simulink model "MSREPrimaryLoop_PlantLevel"  (R2024a)
settings: Solver=VariableStepAuto  StartTime=0.0  StopTime=500000  MaxStep=0.1  RelTol=1e-3
undefined symbols (not defined in the file): a_f, a_g, axialFuelImportance, axialGraphiteImportance, axialPowerFraction, beta, beta_t, bubbleSaturationLevel, bypassRatio, C0, coolantPHXChannelLength, coolantPHXDh, coolantPHXFlowArea, coreCorrectionNominalFlowRate, coreDowncomerArea, coreDowncomerHydraulicDiameter, coreDowncomerLength, coreDowncomerVolume, coreFlowArea, coreFuelVolume, coreInletFlowDistributerArea, coreInletFlowDistributerHydralicDiameter, coreInletFlowDistributerLength, coreInletFlowDistributerVolume, coreLowerPlenumArea, coreLowerPlenumHydraulicDiameter, coreLowerPlenumLength, coreLowerPlenumVolume, coreUpperPlenumArea, coreUpperPlenumLength, coreUpperPlenumVolume, coreVolume, cpGraphite, day, decayScale, decaySSFraction, dissolusionRatio, dMin, dScale, dsmConst, DXeG, externalReactivity, Fiss_factor, fuelChannelHydrualicDiameter, fuelChannelLength, fuelDepositRatio, fuelFraction, fuelGraphiteArea, fuelGraphiteHeatTransferCoefficient, gamma0, gamma1, gamma2, gasExchangeRatio, gasMixingEfficiency, gasPurgeRate, gasStrippingEfficiency, graphiteKDiff, graphiteUnitCellThickness, initialIodineConcentration, InitialXeMolarConcentration ... (+66)
libraries: fl_lib x291, nesl_utility x101, SimscapeFluids_lib x24, simulink x5, slpidlib x1
(part 10 of 13)

== system MSREPrimaryLoop_PlantLevel/Pump MSRE/Pump/PumpIdeal/XenonCalcPump/InterphaseTranfser ==
  note: This local to volume isn't strick. Either add an integral or reduce the length of the node if variation is large.
  CxSalt : Inport
  GasRef : Inport  Port=2
  CxGas : Inport  Port=3
  Constitutive : Subsystem
  MixtureVolume : Gain  Gain=PipeVolume
  Subsystem1 : Subsystem  ReferencedSubsystem=GasToAlpha
  Transfer Term : MATLAB Function  TreatAsAtomicUnit=on
  Ref : PMIOPort  Side=Left
  TranfserRate : Outport
  wires:
  Transfer Term/1(volRate) -> MixtureVolume/1
  MixtureVolume/1 -> TranfserRate/1
  Constitutive/3(k) -> Transfer Term/6(k)
  Constitutive/2(dsm) -> Transfer Term/5(dsm)
  GasRef/1 -> Subsystem1/1
  Subsystem1/1 -> Transfer Term/3(alpha)
  Constitutive/1(K) -> Transfer Term/4(K)
  CxSalt/1 -> Transfer Term/1(CxS)
  CxGas/1 -> Transfer Term/2(CxG)
  connections:
  Constitutive/LConn1 -- Ref/RConn1

== system MSREPrimaryLoop_PlantLevel/Pump MSRE/Pump/PumpIdeal/XenonCalcPump/Salt ==
  XeLIn : Inport  PortDimensions=1
  IodineSNumberDensity : Inport  Port=2  PortDimensions=1
  T_f_ave : Inport  Port=3
  GasRef : Inport  Port=4  PortDimensions=1
  VolumeRate : Inport  Port=5
  Interphase : Inport  Port=6
  Add : Sum  Inputs=+++--  InputSameDT=on
  Decay : Gain  Gain=xeDecayConstant
  InPipeGeneration : Subsystem
      settings: PortSchema="{\"entries\":[{\"content\":{\"sides\":[{\"content\":{\"connectorIds\":[\"In1\"]},\"type\":\"ConnectorPlacement.EquallySpacedRectSide\",\"uuid\":\"cf58f9e2-4051-4ec0-bfd5-a375f3464f67\"},{\"content\":{\"connectorIds\":[\"Out1\"],\"side\":\"RIGHT\"},\"type\":\"ConnectorPlacement.EquallySpacedRectSide\",\"uuid\":\"cf475b22-0422-4ebc-b148-ab559744c6ba\"},{\"content\":{\"connectorIds\":[],\"side\":\"TOP\"},\"type\":\"ConnectorPlacement.EquallySpacedRectSide\",\"uuid\":\"15cc78ce-ee79-4f49-b098-b77c0b2a8ba1\"},{\"content\":{\"connectorIds\":[\"In2\"],\"side\":\"BOTTOM\"},\"type\":\"ConnectorPlacement.EquallySpacedRectSide\",\"uuid\":\"64f5be1f-19d6-4b5f-ac24-c41659a6a539\"}]},\"type\":\"ConnectorPlacement.EquallySpacedConnector\",\"uuid\":\"1fb1607a-ceed-4d70-a511-7b706be0d7ea\"}],\"packageUris\":[\"http://schema.mathworks.com/mf0/Connector/R2020b\"],\"version\":\"1.0\"}"
  LiquidFlowRate : Product
  LiquidVolume : Product  Inputs=*/
  MixtureVolume : Gain  Gain=1/PipeVolume
  PhaseMass : Integrator  LimitOutput=on  LowerSaturationLimit=0
  Subsystem1 : Subsystem
  XeLOut : Outport  PortDimensions=1
  CxSalt : Outport  Port=2
  wires:
  LiquidFlowRate/1 -> Add/5, XeLOut/1
  IodineSNumberDensity/1 -> InPipeGeneration/1(IodineSNumberDensity)
  LiquidVolume/1 -> CxSalt/1, LiquidFlowRate/2
  Add/1 -> PhaseMass/1
  MixtureVolume/1 -> LiquidVolume/1
  VolumeRate/1 -> LiquidFlowRate/1
  T_f_ave/1 -> InPipeGeneration/2(T_f_ave)
  PhaseMass/1 -> Decay/1, MixtureVolume/1
  GasRef/1 -> Subsystem1/1(Gas)
  Subsystem1/1(1-alpha) -> LiquidVolume/2
  InPipeGeneration/1("XenonGenerationRate, [kg/s]") -> Add/2
  XeLIn/1 -> Add/1
  Interphase/1 -> Add/3
  Decay/1 -> Add/4

== system MSREPrimaryLoop_PlantLevel/Pump MSRE/Pump/PumpPysical/PumpPhysics&Control/Pump Drive Control ==
  KI : fl_lib/Physical Signals/Functions/PS Gain  gain=1 1/s
  KP : fl_lib/Physical Signals/Functions/PS Gain  gain=1
  PS Add : fl_lib/Physical Signals/Functions/PS Add
  PS Constant : fl_lib/Physical Signals/Sources/PS Constant  constant=1
  PS Constant1 : fl_lib/Physical Signals/Sources/PS Constant  constant=v_dot m^3/s
  PS Constant2 : fl_lib/Physical Signals/Sources/PS Constant  constant=1 + bypassRatio
  PS Divide : fl_lib/Physical Signals/Functions/PS Divide
  PS Gain : fl_lib/Physical Signals/Functions/PS Gain  gain=2500 rpm
  PS Integrator : fl_lib/Physical Signals/Linear Operators/PS Integrator  reset_method=foundation.enum.IntegratorResetSpec.None  initial_condition_spec=foundation.enum.IntegratorICSpec.Internal  saturation_spec=foundation.enum.IntegratorSaturationSpec.None  saturation_source_spec=foundation.enum.IntegratorSaturationSourceSpec.Internal  x0=1  xu=inf s  xl=-inf s
  PS Product : fl_lib/Physical Signals/Functions/PS Product
  PS Product2 : fl_lib/Physical Signals/Functions/PS Product
  PS Ramp : fl_lib/Physical Signals/Sources/PS Ramp  slope=0.01 1/s  start_time=0 s  initial_output=0.1
  PS Saturation : fl_lib/Physical Signals/Nonlinear Operators/PS Saturation  upper_limit=1  lower_limit=0
  PS Subtract : fl_lib/Physical Signals/Functions/PS Subtract
  RPM : PMIOPort  Side=Left
  VolumeRate : PMIOPort  Port=2  Side=Left
  FlowRef : PMIOPort  Port=3  Side=Right
  connections:
  PS Product2/RConn1 -- PS Gain/LConn1
  PS Product2/LConn2 -- PS Saturation/RConn1
  PS Constant/RConn1 -- PS Product2/LConn1
  PS Ramp/RConn1 -- PS Saturation/LConn1
  PS Divide/LConn1 -- VolumeRate/RConn1
  PS Constant1/RConn1 -- PS Divide/LConn2
  PS Constant2/RConn1 -- PS Subtract/LConn1
  PS Divide/RConn1 -- PS Subtract/LConn2
  KI/LConn1 -- KP/LConn1 -- PS Subtract/RConn1
  KI/RConn1 -- PS Integrator/LConn1
  PS Add/LConn1 -- PS Integrator/RConn1
  KP/RConn1 -- PS Add/LConn2
  PS Gain/RConn1 -- PS Product/LConn1
  PS Add/RConn1 -- PS Product/LConn2
  RPM/RConn1 -- PS Product/RConn1

== system MSREPrimaryLoop_PlantLevel/Pump MSRE/Pump Bowl/Salt Space/XenonCalcBowl/Gas ==
  Interphase : Inport
  VolumeRate : Inport  Port=2
  GasRef : Inport  Port=3
  XeGIn : Inport  Port=4
  Add : Sum  Inputs=+---
  Add1 : Sum  Inputs=+-
  Constant : Constant
  Constant1 : Constant  Value=0.001
  Divide : Product  Inputs=*/
  Gain2 : Gain  Gain=xeDecayConstant
  LiquidFlowRate : Product
  LiquidVolume : Product  Inputs=*/
  MixtureVolume : Gain  Gain=1/PipeVolume
  PhaseMass : Integrator  LimitOutput=on  LowerSaturationLimit=0
  PreventDivideByZero : MinMax  Function=max  Inputs=2
  CxGas : Outport
  XeGOut : Outport  Port=2
  wires:
  LiquidFlowRate/1 -> XeGOut/1, Add/3
  LiquidVolume/1 -> LiquidFlowRate/2
  Add/1 -> PhaseMass/1
  Constant/1 -> Add1/1
  MixtureVolume/1 -> Divide/1, LiquidVolume/1
  Add1/1 -> LiquidVolume/2
  VolumeRate/1 -> LiquidFlowRate/1
  XeGIn/1 -> Add/1
  Gain2/1 -> Add/4
  PhaseMass/1 -> Gain2/1, MixtureVolume/1
  Interphase/1 -> Add/2
  PreventDivideByZero/1 -> Divide/2
  Constant1/1 -> PreventDivideByZero/2
  Divide/1 -> CxGas/1
  GasRef/1 -> Add1/2, PreventDivideByZero/1

== system MSREPrimaryLoop_PlantLevel/Pump MSRE/Pump Bowl/Salt Space/XenonCalcBowl/InterphaseTranfser ==
  note: This local to volume isn't strick. Either add an integral or reduce the length of the node if variation is large.
  CxSalt : Inport
  GasRef : Inport  Port=2
  CxGas : Inport  Port=3
  Constitutive : Subsystem
  MixtureVolume : Gain  Gain=PipeVolume
  Transfer Term : MATLAB Function  TreatAsAtomicUnit=on
  Ref : PMIOPort  Side=Left
  TranfserRate : Outport
  wires:
  Transfer Term/1(volRate) -> MixtureVolume/1
  MixtureVolume/1 -> TranfserRate/1
  Constitutive/3(k) -> Transfer Term/6(k)
  Constitutive/2(dsm) -> Transfer Term/5(dsm)
  Constitutive/1(K) -> Transfer Term/4(K)
  CxSalt/1 -> Transfer Term/1(CxS)
  CxGas/1 -> Transfer Term/2(CxG)
  GasRef/1 -> Transfer Term/3(alpha)
  connections:
  Constitutive/LConn1 -- Ref/RConn1

== system MSREPrimaryLoop_PlantLevel/Pump MSRE/Pump Bowl/Salt Space/XenonCalcBowl/Salt ==
  XeLIn : Inport  PortDimensions=1
  IodineSNumberDensity : Inport  Port=2  PortDimensions=1
  T_f_ave : Inport  Port=3
  GasRef : Inport  Port=4  PortDimensions=1
  VolumeRate : Inport  Port=5
  Interphase : Inport  Port=6
  Add : Sum  Inputs=+++--  InputSameDT=on
  Decay : Gain  Gain=xeDecayConstant
  InPipeGeneration : Subsystem
      settings: PortSchema="{\"entries\":[{\"content\":{\"sides\":[{\"content\":{\"connectorIds\":[\"In1\"]},\"type\":\"ConnectorPlacement.EquallySpacedRectSide\",\"uuid\":\"cf58f9e2-4051-4ec0-bfd5-a375f3464f67\"},{\"content\":{\"connectorIds\":[\"Out1\"],\"side\":\"RIGHT\"},\"type\":\"ConnectorPlacement.EquallySpacedRectSide\",\"uuid\":\"cf475b22-0422-4ebc-b148-ab559744c6ba\"},{\"content\":{\"connectorIds\":[],\"side\":\"TOP\"},\"type\":\"ConnectorPlacement.EquallySpacedRectSide\",\"uuid\":\"15cc78ce-ee79-4f49-b098-b77c0b2a8ba1\"},{\"content\":{\"connectorIds\":[\"In2\"],\"side\":\"BOTTOM\"},\"type\":\"ConnectorPlacement.EquallySpacedRectSide\",\"uuid\":\"64f5be1f-19d6-4b5f-ac24-c41659a6a539\"}]},\"type\":\"ConnectorPlacement.EquallySpacedConnector\",\"uuid\":\"1fb1607a-ceed-4d70-a511-7b706be0d7ea\"}],\"packageUris\":[\"http://schema.mathworks.com/mf0/Connector/R2020b\"],\"version\":\"1.0\"}"
  LiquidFlowRate : Product
  LiquidVolume : Product  Inputs=*/
  MixtureVolume : Gain  Gain=1/PipeVolume
  PhaseMass : Integrator  LimitOutput=on  LowerSaturationLimit=0
  Subsystem1 : Subsystem
  XeLOut : Outport  PortDimensions=1
  CxSalt : Outport  Port=2
  wires:
  LiquidFlowRate/1 -> Add/5, XeLOut/1
  IodineSNumberDensity/1 -> InPipeGeneration/1(IodineSNumberDensity)
  LiquidVolume/1 -> CxSalt/1, LiquidFlowRate/2
  Add/1 -> PhaseMass/1
  MixtureVolume/1 -> LiquidVolume/1
  VolumeRate/1 -> LiquidFlowRate/1
  T_f_ave/1 -> InPipeGeneration/2(T_f_ave)
  PhaseMass/1 -> Decay/1, MixtureVolume/1
  GasRef/1 -> Subsystem1/1(Gas)
  Subsystem1/1(1-alpha) -> LiquidVolume/2
  InPipeGeneration/1("XenonGenerationRate, [kg/s]") -> Add/2
  XeLIn/1 -> Add/1
  Interphase/1 -> Add/3
  Decay/1 -> Add/4

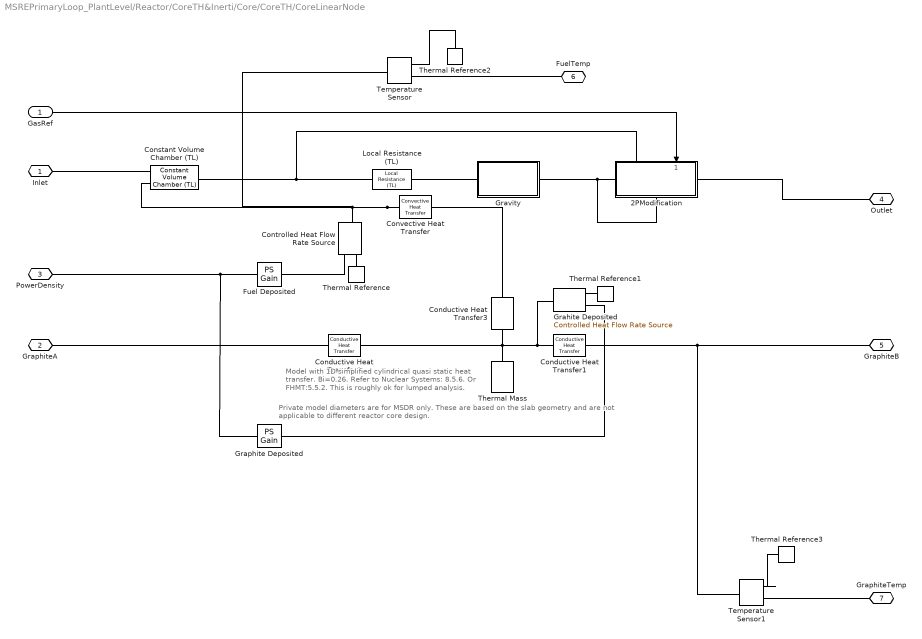
== system MSREPrimaryLoop_PlantLevel/Reactor/CoreTH&Inerti/Core/CoreTH/CoreLinearNode ==
  note: Private model diameters are for MSDR only. These are based on the slab geometry and are not applicable to different reactor core design.
  note: Model with 1D simplified cylindrical quasi static heat transfer. Bi=0.26.
      | Refer to Nuclear Systems: 8.5.6. Or FHMT:5.5.2.
      | This is roughly ok for lumped analysis.
  GasRef : Inport
  2PModification : Subsystem  ReferencedSubsystem=TwoPhaseModification
      settings: PortSchema="{\"entries\":[{\"content\":{\"sides\":[{\"content\":{\"connectorIds\":[\"LConn1\"]},\"type\":\"ConnectorPlacement.EquallySpacedRectSide\",\"uuid\":\"7546b4b7-b669-49c8-8f27-f696391ea3ad\"},{\"content\":{\"connectorIds\":[\"RConn1\"],\"side\":\"RIGHT\"},\"type\":\"ConnectorPlacement.EquallySpacedRectSide\",\"uuid\":\"0e6176f2-177c-4327-bcfa-9a190fe9083f\"},{\"content\":{\"connectorIds\":[\"LConn2\",\"In1\"],\"side\":\"TOP\"},\"type\":\"ConnectorPlacement.EquallySpacedRectSide\",\"uuid\":\"16faf74c-4635-4009-a5b3-33dd03b625c6\"},{\"content\":{\"connectorIds\":[\"RConn2\"],\"side\":\"BOTTOM\"},\"type\":\"ConnectorPlacement.EquallySpacedRectSide\",\"uuid\":\"2081d73b-bb08-4ad9-b5c8-e48a4e9c4e20\"}]},\"type\":\"ConnectorPlacement.EquallySpacedConnector\",\"uuid\":\"243e4075-206b-4747-a8bc-b8f10d9a577f\"}],\"packageUris\":[\"http://schema.mathworks.com/mf0/Connector/R2020b\"],\"version\":\"1.0\"}"
  Conductive Heat Transfer1 : fl_lib/Thermal/Thermal Elements/Conductive Heat Transfer  thermal_type=foundation.enum.ConstantVariableTabulated.Constant  wall_geometry=foundation.enum.ConductionWallGeometry.Planar  area=CoreVolume/CoreLength*(1-FuelFraction) m^2  thickness=0.5*CoreLength/N_nodes m  d_in=0.05 m  d_out=0.1 m  L=1 m  th_cond_min=10 W/(K*m)  th_cond=k_graphite W/(m*K)  th_cond_TLU=[413, 401, 392, 383, 371, 357, 342] W/(K*m)  temp_TLU=[200, 273, 400, 600, 800, 1000, 1200] K  T_specify=off  T_priority=None  T=0 K  T_nominal_specify=off  T_nominal_value=1  T_nominal_unit=K  Q_specify=off  Q_priority=None  Q=0 W  Q_nominal_specify=off  Q_nominal_value=1  Q_nominal_unit=W
  Conductive Heat Transfer2 : fl_lib/Thermal/Thermal Elements/Conductive Heat Transfer  thermal_type=foundation.enum.ConstantVariableTabulated.Constant  wall_geometry=foundation.enum.ConductionWallGeometry.Planar  area=CoreVolume/CoreLength*(1-FuelFraction) m^2  thickness=0.5*CoreLength/N_nodes m  d_in=0.05 m  d_out=0.1 m  L=1 m  th_cond_min=10 W/(K*m)  th_cond=k_graphite W/(m*K)  th_cond_TLU=[413, 401, 392, 383, 371, 357, 342] W/(K*m)  temp_TLU=[200, 273, 400, 600, 800, 1000, 1200] K  T_specify=off  T_priority=None  T=0 K  T_nominal_specify=off  T_nominal_value=1  T_nominal_unit=K  Q_specify=off  Q_priority=None  Q=0 W  Q_nominal_specify=off  Q_nominal_value=1  Q_nominal_unit=W
  Conductive Heat Transfer3 : fl_lib/Thermal/Thermal Elements/Conductive Heat Transfer  thermal_type=foundation.enum.ConstantVariableTabulated.Constant  wall_geometry=foundation.enum.ConductionWallGeometry.Planar  area=FuelGraphiteArea/N_nodes m^2  thickness=0.5*UnitCellGraphiteThickness m  d_in=0.05 m  d_out=0.1 m  L=1 m  th_cond_min=10 W/(K*m)  th_cond=k_graphite W/(m*K)  th_cond_TLU=[413, 401, 392, 383, 371, 357, 342] W/(K*m)  temp_TLU=[200, 273, 400, 600, 800, 1000, 1200] K  T_specify=off  T_priority=None  T=0 K  T_nominal_specify=off  T_nominal_value=1  T_nominal_unit=K  Q_specify=off  Q_priority=None  Q=0 W  Q_nominal_specify=off  Q_nominal_value=1  Q_nominal_unit=W
  Constant Volume Chamber (TL) : fl_lib/Thermal Liquid/Elements/Constant Volume Chamber (TL)  volume=coreFuelVolume/N_nodes m^3  num_ports=foundation.enum.num_ports.two  area_A=coreFlowArea m^2  area_B=coreFlowArea m^2  area_C=0.01 m^2  area_D=0.01 m^2  p_I_specify=on  p_I_priority=None  p_I=P0 Pa  p_I_nominal_specify=off  p_I_nominal_value=1  p_I_nominal_unit=MPa  T_I_specify=on  T_I_priority=None  T_I=T0 K  T_I_nominal_specify=on  T_I_nominal_value=T0  T_I_nominal_unit=K  u_I_specify=on  u_I_priority=None  u_I=cpMSRE J/kg  u_I_nominal_specify=off  u_I_nominal_value=1  u_I_nominal_unit=kJ/kg  rho_I_specify=on  rho_I_priority=None  rho_I=nominalFuelDensity kg/m^3  rho_I_nominal_specify=off  rho_I_nominal_value=1  rho_I_nominal_unit=kg/m^3
      settings: LogSimulationData=on  InternalSimscapePortConfiguration="{\"Bottom\":[],\"Left\":[{\"id\":\"A\",\"label\":\"A\",\"type\":\"foundation.thermal_liquid.thermal_liquid\"},{\"id\":\"H\",\"label\":\"H\",\"type\":\"foundation.thermal.thermal\"}],\"Right\":[{\"id\":\"B\",\"label\":\"B\",\"type\":\"foundation.thermal_liquid.thermal_liquid\"}],\"Top\":[]}"
  Controlled Heat Flow Rate Source : fl_lib/Thermal/Thermal Sources/Controlled Heat Flow Rate Source
      settings: LogSimulationData=on
  Convective Heat Transfer : fl_lib/Thermal/Thermal Elements/Convective Heat Transfer  thermal_type=foundation.enum.constant_variable.constant  area=fuelGraphiteArea/N_nodes m^2  heat_tr_coeff=fuelGraphiteHeatTransferCoefficient W/(K*m^2)  min_heat_tr_coeff=1e-3 W/(K*m^2)  T_specify=off  T_priority=None  T=0 K  T_nominal_specify=off  T_nominal_value=1  T_nominal_unit=K  Q_specify=off  Q_priority=None  Q=0 W  Q_nominal_specify=off  Q_nominal_value=1  Q_nominal_unit=W
  Fuel Deposited : fl_lib/Physical Signals/Functions/PS Gain  gain=FuelDepositRatio*CoreVolume*axialPowerFraction(1) m^3
  Grahite Deposited : fl_lib/Thermal/Thermal Sources/Controlled Heat Flow Rate Source
      settings: LogSimulationData=on
  Graphite Deposited : fl_lib/Physical Signals/Functions/PS Gain  gain=(1-FuelDepositRatio)*CoreVolume*axialPowerFraction(1) m^3
  Gravity : Subsystem
  Local Resistance (TL) : SimscapeFluids_lib/Thermal Liquid/Pipes & Fittings/Local Resistance (TL)  resistance_loss_spec=fluids.thermal_liquid.pipes_fittings.enum.ResistanceLossSpec.Constant  loss_coeff_AB=fuelChannelLength/N_nodes/fuelChannelHydrualicDiameter*0.07  loss_coeff_BA=fuelChannelLength/N_nodes/fuelChannelHydrualicDiameter*0.07  Re_TLU=[-500, -200, -100, -50, -40, -30, -20, -10, 10, 20, 30, 40, 50, 100, 200, 500, 1000, 2000]  loss_coeff_TLU=[.65, .75, .9, 1.15, 1.35, 1.65, 2.3, 3.1, 4, 2.7, 1.8, 1.46, 1.3, .9, .65, .42, .3, .2]  flow_area=coreFlowArea m^2  Re_c=150
      settings: InternalSimscapePortConfiguration="{\"Bottom\":[],\"Left\":[{\"id\":\"A\",\"label\":\"A\",\"type\":\"foundation.thermal_liquid.thermal_liquid\"}],\"Right\":[{\"id\":\"B\",\"label\":\"B\",\"type\":\"foundation.thermal_liquid.thermal_liquid\"}],\"Top\":[]}"
  Temperature Sensor : fl_lib/Thermal/Thermal Sensors/Temperature Sensor  temperature_measure=foundation.enum.MeasurementReference.difference
  Temperature Sensor1 : fl_lib/Thermal/Thermal Sensors/Temperature Sensor  temperature_measure=foundation.enum.MeasurementReference.difference
  Thermal Mass : fl_lib/Thermal/Thermal Elements/Thermal Mass  mass_type=foundation.enum.constant_variable.constant  mass=CoreVolume*(1-FuelFraction)*rho_graphite/N_nodes kg  sp_heat=cp_graphite J/(K*kg)  mass_min=1e-6 kg  num_ports=foundation.enum.numPorts2.one  m_specify=off  m_priority=High  m=1 kg  m_nominal_specify=off  m_nominal_value=1  m_nominal_unit=kg  T_specify=on  T_priority=High  T=T0 K  T_nominal_specify=off  T_nominal_value=1  T_nominal_unit=K  Q_specify=off  Q_priority=None  Q=0 W  Q_nominal_specify=off  Q_nominal_value=1  Q_nominal_unit=W
      settings: LogSimulationData=on
  Thermal Reference{,1..3} (4 alike) : fl_lib/Thermal/Thermal Elements/Thermal Reference
  Inlet : PMIOPort  Side=Left
  GraphiteA : PMIOPort  Port=2  Side=Left
  PowerDensity : PMIOPort  Port=3  Side=Left
  Outlet : PMIOPort  Port=4  Side=Right
  GraphiteB : PMIOPort  Port=5  Side=Right
  FuelTemp : PMIOPort  Port=6  Side=Right
  GraphiteTemp : PMIOPort  Port=7  Side=Right
  wires:
  GasRef/1 -> 2PModification/1
  connections:
  Grahite Deposited/LConn1 -- Conductive Heat Transfer3/RConn1 -- Conductive Heat Transfer2/RConn1 -- Thermal Mass/LConn1 -- Conductive Heat Transfer1/LConn1
  Graphite Deposited/LConn1 -- Fuel Deposited/LConn1 -- PowerDensity/RConn1
  Conductive Heat Transfer1/RConn1 -- Temperature Sensor1/LConn1 -- GraphiteB/RConn1
  Grahite Deposited/RConn1 -- Graphite Deposited/RConn1
  GraphiteA/RConn1 -- Conductive Heat Transfer2/LConn1
  Controlled Heat Flow Rate Source/RConn2 -- Thermal Reference/LConn1
  Grahite Deposited/RConn2 -- Thermal Reference1/LConn1
  Fuel Deposited/RConn1 -- Controlled Heat Flow Rate Source/RConn1
  Outlet/RConn1 -- 2PModification/RConn1
  Temperature Sensor/RConn1 -- Thermal Reference2/LConn1
  Temperature Sensor/RConn2 -- FuelTemp/RConn1
  2PModification/LConn2 -- Constant Volume Chamber (TL)/RConn1 -- Local Resistance (TL)/LConn1
  Inlet/RConn1 -- Constant Volume Chamber (TL)/LConn1
  Gravity/LConn1 -- Local Resistance (TL)/RConn1
  Conductive Heat Transfer3/LConn1 -- Convective Heat Transfer/RConn1
  Convective Heat Transfer/LConn1 -- Constant Volume Chamber (TL)/LConn2 -- Temperature Sensor/LConn1 -- Controlled Heat Flow Rate Source/LConn1
  Temperature Sensor1/RConn2 -- GraphiteTemp/RConn1
  Temperature Sensor1/RConn1 -- Thermal Reference3/LConn1
  2PModification/LConn1 -- 2PModification/RConn2 -- Gravity/RConn1

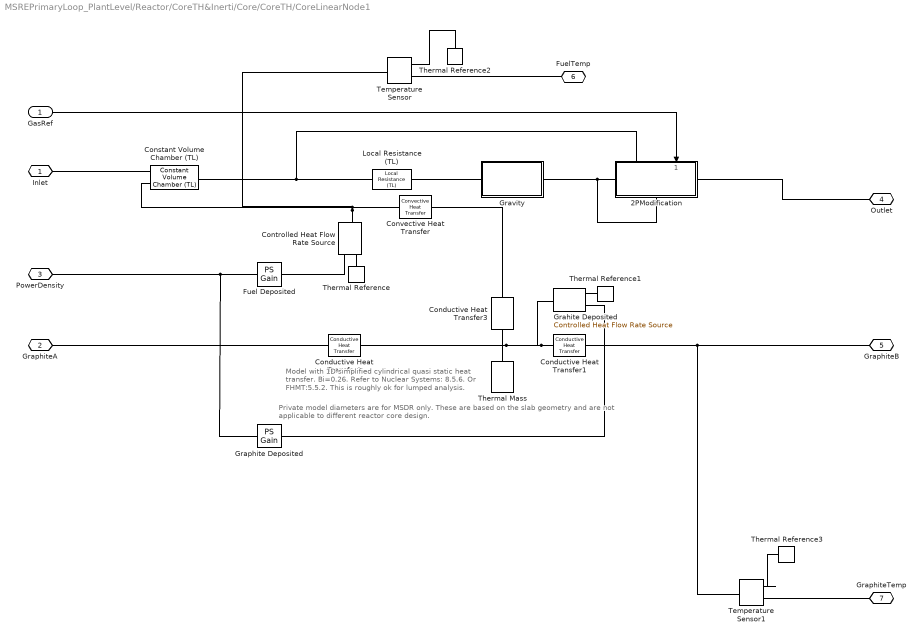
== system MSREPrimaryLoop_PlantLevel/Reactor/CoreTH&Inerti/Core/CoreTH/CoreLinearNode1 ==
  note: Model with 1D simplified cylindrical quasi static heat transfer. Bi=0.26.
      | Refer to Nuclear Systems: 8.5.6. Or FHMT:5.5.2.
      | This is roughly ok for lumped analysis.
  note: Private model diameters are for MSDR only. These are based on the slab geometry and are not applicable to different reactor core design.
  GasRef : Inport
  2PModification : Subsystem  ReferencedSubsystem=TwoPhaseModification
      settings: PortSchema="{\"entries\":[{\"content\":{\"sides\":[{\"content\":{\"connectorIds\":[\"LConn1\"]},\"type\":\"ConnectorPlacement.EquallySpacedRectSide\",\"uuid\":\"7546b4b7-b669-49c8-8f27-f696391ea3ad\"},{\"content\":{\"connectorIds\":[\"RConn1\"],\"side\":\"RIGHT\"},\"type\":\"ConnectorPlacement.EquallySpacedRectSide\",\"uuid\":\"0e6176f2-177c-4327-bcfa-9a190fe9083f\"},{\"content\":{\"connectorIds\":[\"LConn2\",\"In1\"],\"side\":\"TOP\"},\"type\":\"ConnectorPlacement.EquallySpacedRectSide\",\"uuid\":\"16faf74c-4635-4009-a5b3-33dd03b625c6\"},{\"content\":{\"connectorIds\":[\"RConn2\"],\"side\":\"BOTTOM\"},\"type\":\"ConnectorPlacement.EquallySpacedRectSide\",\"uuid\":\"2081d73b-bb08-4ad9-b5c8-e48a4e9c4e20\"}]},\"type\":\"ConnectorPlacement.EquallySpacedConnector\",\"uuid\":\"243e4075-206b-4747-a8bc-b8f10d9a577f\"}],\"packageUris\":[\"http://schema.mathworks.com/mf0/Connector/R2020b\"],\"version\":\"1.0\"}"
  Conductive Heat Transfer1 : fl_lib/Thermal/Thermal Elements/Conductive Heat Transfer  thermal_type=foundation.enum.ConstantVariableTabulated.Constant  wall_geometry=foundation.enum.ConductionWallGeometry.Planar  area=CoreVolume/CoreLength*(1-FuelFraction) m^2  thickness=0.5*CoreLength/N_nodes m  d_in=0.05 m  d_out=0.1 m  L=1 m  th_cond_min=10 W/(K*m)  th_cond=k_graphite W/(m*K)  th_cond_TLU=[413, 401, 392, 383, 371, 357, 342] W/(K*m)  temp_TLU=[200, 273, 400, 600, 800, 1000, 1200] K  T_specify=off  T_priority=None  T=0 K  T_nominal_specify=off  T_nominal_value=1  T_nominal_unit=K  Q_specify=off  Q_priority=None  Q=0 W  Q_nominal_specify=off  Q_nominal_value=1  Q_nominal_unit=W
  Conductive Heat Transfer2 : fl_lib/Thermal/Thermal Elements/Conductive Heat Transfer  thermal_type=foundation.enum.ConstantVariableTabulated.Constant  wall_geometry=foundation.enum.ConductionWallGeometry.Planar  area=CoreVolume/CoreLength*(1-FuelFraction) m^2  thickness=0.5*CoreLength/N_nodes m  d_in=0.05 m  d_out=0.1 m  L=1 m  th_cond_min=10 W/(K*m)  th_cond=k_graphite W/(m*K)  th_cond_TLU=[413, 401, 392, 383, 371, 357, 342] W/(K*m)  temp_TLU=[200, 273, 400, 600, 800, 1000, 1200] K  T_specify=off  T_priority=None  T=0 K  T_nominal_specify=off  T_nominal_value=1  T_nominal_unit=K  Q_specify=off  Q_priority=None  Q=0 W  Q_nominal_specify=off  Q_nominal_value=1  Q_nominal_unit=W
  Conductive Heat Transfer3 : fl_lib/Thermal/Thermal Elements/Conductive Heat Transfer  thermal_type=foundation.enum.ConstantVariableTabulated.Constant  wall_geometry=foundation.enum.ConductionWallGeometry.Planar  area=FuelGraphiteArea/N_nodes m^2  thickness=0.5*UnitCellGraphiteThickness m  d_in=0.05 m  d_out=0.1 m  L=1 m  th_cond_min=10 W/(K*m)  th_cond=k_graphite W/(m*K)  th_cond_TLU=[413, 401, 392, 383, 371, 357, 342] W/(K*m)  temp_TLU=[200, 273, 400, 600, 800, 1000, 1200] K  T_specify=off  T_priority=None  T=0 K  T_nominal_specify=off  T_nominal_value=1  T_nominal_unit=K  Q_specify=off  Q_priority=None  Q=0 W  Q_nominal_specify=off  Q_nominal_value=1  Q_nominal_unit=W
  Constant Volume Chamber (TL) : fl_lib/Thermal Liquid/Elements/Constant Volume Chamber (TL)  volume=coreFuelVolume/N_nodes m^3  num_ports=foundation.enum.num_ports.two  area_A=coreFlowArea m^2  area_B=coreFlowArea m^2  area_C=0.01 m^2  area_D=0.01 m^2  p_I_specify=on  p_I_priority=None  p_I=P0 Pa  p_I_nominal_specify=off  p_I_nominal_value=1  p_I_nominal_unit=MPa  T_I_specify=on  T_I_priority=None  T_I=T0 K  T_I_nominal_specify=on  T_I_nominal_value=T0  T_I_nominal_unit=K  u_I_specify=on  u_I_priority=None  u_I=cpMSRE J/kg  u_I_nominal_specify=off  u_I_nominal_value=1  u_I_nominal_unit=kJ/kg  rho_I_specify=on  rho_I_priority=None  rho_I=nominalFuelDensity kg/m^3  rho_I_nominal_specify=off  rho_I_nominal_value=1  rho_I_nominal_unit=kg/m^3
      settings: LogSimulationData=on  InternalSimscapePortConfiguration="{\"Bottom\":[],\"Left\":[{\"id\":\"A\",\"label\":\"A\",\"type\":\"foundation.thermal_liquid.thermal_liquid\"},{\"id\":\"H\",\"label\":\"H\",\"type\":\"foundation.thermal.thermal\"}],\"Right\":[{\"id\":\"B\",\"label\":\"B\",\"type\":\"foundation.thermal_liquid.thermal_liquid\"}],\"Top\":[]}"
  Controlled Heat Flow Rate Source : fl_lib/Thermal/Thermal Sources/Controlled Heat Flow Rate Source
      settings: LogSimulationData=on
  Convective Heat Transfer : fl_lib/Thermal/Thermal Elements/Convective Heat Transfer  thermal_type=foundation.enum.constant_variable.constant  area=fuelGraphiteArea/N_nodes m^2  heat_tr_coeff=fuelGraphiteHeatTransferCoefficient W/(K*m^2)  min_heat_tr_coeff=1e-3 W/(K*m^2)  T_specify=off  T_priority=None  T=0 K  T_nominal_specify=off  T_nominal_value=1  T_nominal_unit=K  Q_specify=off  Q_priority=None  Q=0 W  Q_nominal_specify=off  Q_nominal_value=1  Q_nominal_unit=W
  Fuel Deposited : fl_lib/Physical Signals/Functions/PS Gain  gain=FuelDepositRatio*CoreVolume*axialPowerFraction(2) m^3
  Grahite Deposited : fl_lib/Thermal/Thermal Sources/Controlled Heat Flow Rate Source
      settings: LogSimulationData=on
  Graphite Deposited : fl_lib/Physical Signals/Functions/PS Gain  gain=(1-FuelDepositRatio)*CoreVolume*axialPowerFraction(2) m^3
  Gravity : Subsystem
  Local Resistance (TL) : SimscapeFluids_lib/Thermal Liquid/Pipes & Fittings/Local Resistance (TL)  resistance_loss_spec=fluids.thermal_liquid.pipes_fittings.enum.ResistanceLossSpec.Constant  loss_coeff_AB=fuelChannelLength/N_nodes/fuelChannelHydrualicDiameter*0.07  loss_coeff_BA=fuelChannelLength/N_nodes/fuelChannelHydrualicDiameter*0.07  Re_TLU=[-500, -200, -100, -50, -40, -30, -20, -10, 10, 20, 30, 40, 50, 100, 200, 500, 1000, 2000]  loss_coeff_TLU=[.65, .75, .9, 1.15, 1.35, 1.65, 2.3, 3.1, 4, 2.7, 1.8, 1.46, 1.3, .9, .65, .42, .3, .2]  flow_area=coreFlowArea m^2  Re_c=150
      settings: InternalSimscapePortConfiguration="{\"Bottom\":[],\"Left\":[{\"id\":\"A\",\"label\":\"A\",\"type\":\"foundation.thermal_liquid.thermal_liquid\"}],\"Right\":[{\"id\":\"B\",\"label\":\"B\",\"type\":\"foundation.thermal_liquid.thermal_liquid\"}],\"Top\":[]}"
  Temperature Sensor : fl_lib/Thermal/Thermal Sensors/Temperature Sensor  temperature_measure=foundation.enum.MeasurementReference.difference
  Temperature Sensor1 : fl_lib/Thermal/Thermal Sensors/Temperature Sensor  temperature_measure=foundation.enum.MeasurementReference.difference
  Thermal Mass : fl_lib/Thermal/Thermal Elements/Thermal Mass  mass_type=foundation.enum.constant_variable.constant  mass=CoreVolume*(1-FuelFraction)*rho_graphite/N_nodes kg  sp_heat=cp_graphite J/(K*kg)  mass_min=1e-6 kg  num_ports=foundation.enum.numPorts2.one  m_specify=off  m_priority=High  m=1 kg  m_nominal_specify=off  m_nominal_value=1  m_nominal_unit=kg  T_specify=on  T_priority=High  T=T0 K  T_nominal_specify=off  T_nominal_value=1  T_nominal_unit=K  Q_specify=off  Q_priority=None  Q=0 W  Q_nominal_specify=off  Q_nominal_value=1  Q_nominal_unit=W
      settings: LogSimulationData=on
  Thermal Reference{,1..3} (4 alike) : fl_lib/Thermal/Thermal Elements/Thermal Reference
  Inlet : PMIOPort  Side=Left
  GraphiteA : PMIOPort  Port=2  Side=Left
  PowerDensity : PMIOPort  Port=3  Side=Left
  Outlet : PMIOPort  Port=4  Side=Right
  GraphiteB : PMIOPort  Port=5  Side=Right
  FuelTemp : PMIOPort  Port=6  Side=Right
  GraphiteTemp : PMIOPort  Port=7  Side=Right
  wires:
  GasRef/1 -> 2PModification/1
  connections:
  Temperature Sensor1/RConn1 -- Thermal Reference3/LConn1
  Temperature Sensor1/RConn2 -- GraphiteTemp/RConn1
  Controlled Heat Flow Rate Source/LConn1 -- Temperature Sensor/LConn1 -- Constant Volume Chamber (TL)/LConn2 -- Convective Heat Transfer/LConn1
  Conductive Heat Transfer3/LConn1 -- Convective Heat Transfer/RConn1
  Gravity/LConn1 -- Local Resistance (TL)/RConn1
  Inlet/RConn1 -- Constant Volume Chamber (TL)/LConn1
  Local Resistance (TL)/LConn1 -- Constant Volume Chamber (TL)/RConn1 -- 2PModification/LConn2
  Temperature Sensor/RConn2 -- FuelTemp/RConn1
  Temperature Sensor/RConn1 -- Thermal Reference2/LConn1
  Outlet/RConn1 -- 2PModification/RConn1
  Fuel Deposited/RConn1 -- Controlled Heat Flow Rate Source/RConn1
  Grahite Deposited/RConn2 -- Thermal Reference1/LConn1
  Controlled Heat Flow Rate Source/RConn2 -- Thermal Reference/LConn1
  GraphiteA/RConn1 -- Conductive Heat Transfer2/LConn1
  Grahite Deposited/RConn1 -- Graphite Deposited/RConn1
  Temperature Sensor1/LConn1 -- Conductive Heat Transfer1/RConn1 -- GraphiteB/RConn1
  PowerDensity/RConn1 -- Fuel Deposited/LConn1 -- Graphite Deposited/LConn1
  Conductive Heat Transfer1/LConn1 -- Thermal Mass/LConn1 -- Conductive Heat Transfer2/RConn1 -- Conductive Heat Transfer3/RConn1 -- Grahite Deposited/LConn1
  2PModification/LConn1 -- Gravity/RConn1 -- 2PModification/RConn2

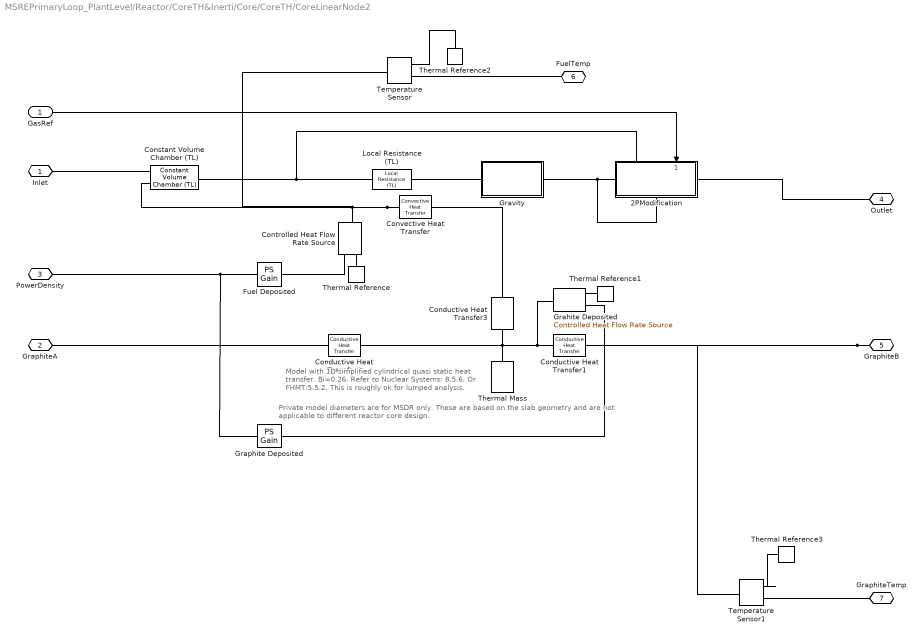
== system MSREPrimaryLoop_PlantLevel/Reactor/CoreTH&Inerti/Core/CoreTH/CoreLinearNode2 ==
  note: Private model diameters are for MSDR only. These are based on the slab geometry and are not applicable to different reactor core design.
  note: Model with 1D simplified cylindrical quasi static heat transfer. Bi=0.26.
      | Refer to Nuclear Systems: 8.5.6. Or FHMT:5.5.2.
      | This is roughly ok for lumped analysis.
  GasRef : Inport
  2PModification : Subsystem  ReferencedSubsystem=TwoPhaseModification
      settings: PortSchema="{\"entries\":[{\"content\":{\"sides\":[{\"content\":{\"connectorIds\":[\"LConn1\"]},\"type\":\"ConnectorPlacement.EquallySpacedRectSide\",\"uuid\":\"7546b4b7-b669-49c8-8f27-f696391ea3ad\"},{\"content\":{\"connectorIds\":[\"RConn1\"],\"side\":\"RIGHT\"},\"type\":\"ConnectorPlacement.EquallySpacedRectSide\",\"uuid\":\"0e6176f2-177c-4327-bcfa-9a190fe9083f\"},{\"content\":{\"connectorIds\":[\"LConn2\",\"In1\"],\"side\":\"TOP\"},\"type\":\"ConnectorPlacement.EquallySpacedRectSide\",\"uuid\":\"16faf74c-4635-4009-a5b3-33dd03b625c6\"},{\"content\":{\"connectorIds\":[\"RConn2\"],\"side\":\"BOTTOM\"},\"type\":\"ConnectorPlacement.EquallySpacedRectSide\",\"uuid\":\"2081d73b-bb08-4ad9-b5c8-e48a4e9c4e20\"}]},\"type\":\"ConnectorPlacement.EquallySpacedConnector\",\"uuid\":\"243e4075-206b-4747-a8bc-b8f10d9a577f\"}],\"packageUris\":[\"http://schema.mathworks.com/mf0/Connector/R2020b\"],\"version\":\"1.0\"}"
  Conductive Heat Transfer1 : fl_lib/Thermal/Thermal Elements/Conductive Heat Transfer  thermal_type=foundation.enum.ConstantVariableTabulated.Constant  wall_geometry=foundation.enum.ConductionWallGeometry.Planar  area=CoreVolume/CoreLength*(1-FuelFraction) m^2  thickness=0.5*CoreLength/N_nodes m  d_in=0.05 m  d_out=0.1 m  L=1 m  th_cond_min=10 W/(K*m)  th_cond=k_graphite W/(m*K)  th_cond_TLU=[413, 401, 392, 383, 371, 357, 342] W/(K*m)  temp_TLU=[200, 273, 400, 600, 800, 1000, 1200] K  T_specify=off  T_priority=None  T=0 K  T_nominal_specify=off  T_nominal_value=1  T_nominal_unit=K  Q_specify=off  Q_priority=None  Q=0 W  Q_nominal_specify=off  Q_nominal_value=1  Q_nominal_unit=W
  Conductive Heat Transfer2 : fl_lib/Thermal/Thermal Elements/Conductive Heat Transfer  thermal_type=foundation.enum.ConstantVariableTabulated.Constant  wall_geometry=foundation.enum.ConductionWallGeometry.Planar  area=CoreVolume/CoreLength*(1-FuelFraction) m^2  thickness=0.5*CoreLength/N_nodes m  d_in=0.05 m  d_out=0.1 m  L=1 m  th_cond_min=10 W/(K*m)  th_cond=k_graphite W/(m*K)  th_cond_TLU=[413, 401, 392, 383, 371, 357, 342] W/(K*m)  temp_TLU=[200, 273, 400, 600, 800, 1000, 1200] K  T_specify=off  T_priority=None  T=0 K  T_nominal_specify=off  T_nominal_value=1  T_nominal_unit=K  Q_specify=off  Q_priority=None  Q=0 W  Q_nominal_specify=off  Q_nominal_value=1  Q_nominal_unit=W
  Conductive Heat Transfer3 : fl_lib/Thermal/Thermal Elements/Conductive Heat Transfer  thermal_type=foundation.enum.ConstantVariableTabulated.Constant  wall_geometry=foundation.enum.ConductionWallGeometry.Planar  area=FuelGraphiteArea/N_nodes m^2  thickness=0.5*UnitCellGraphiteThickness m  d_in=0.05 m  d_out=0.1 m  L=1 m  th_cond_min=10 W/(K*m)  th_cond=k_graphite W/(m*K)  th_cond_TLU=[413, 401, 392, 383, 371, 357, 342] W/(K*m)  temp_TLU=[200, 273, 400, 600, 800, 1000, 1200] K  T_specify=off  T_priority=None  T=0 K  T_nominal_specify=off  T_nominal_value=1  T_nominal_unit=K  Q_specify=off  Q_priority=None  Q=0 W  Q_nominal_specify=off  Q_nominal_value=1  Q_nominal_unit=W
  Constant Volume Chamber (TL) : fl_lib/Thermal Liquid/Elements/Constant Volume Chamber (TL)  volume=coreFuelVolume/N_nodes m^3  num_ports=foundation.enum.num_ports.two  area_A=coreFlowArea m^2  area_B=coreFlowArea m^2  area_C=0.01 m^2  area_D=0.01 m^2  p_I_specify=on  p_I_priority=None  p_I=P0 Pa  p_I_nominal_specify=off  p_I_nominal_value=1  p_I_nominal_unit=MPa  T_I_specify=on  T_I_priority=None  T_I=T0 K  T_I_nominal_specify=on  T_I_nominal_value=T0  T_I_nominal_unit=K  u_I_specify=on  u_I_priority=None  u_I=cpMSRE J/kg  u_I_nominal_specify=off  u_I_nominal_value=1  u_I_nominal_unit=kJ/kg  rho_I_specify=on  rho_I_priority=None  rho_I=nominalFuelDensity kg/m^3  rho_I_nominal_specify=off  rho_I_nominal_value=1  rho_I_nominal_unit=kg/m^3
      settings: LogSimulationData=on  InternalSimscapePortConfiguration="{\"Bottom\":[],\"Left\":[{\"id\":\"A\",\"label\":\"A\",\"type\":\"foundation.thermal_liquid.thermal_liquid\"},{\"id\":\"H\",\"label\":\"H\",\"type\":\"foundation.thermal.thermal\"}],\"Right\":[{\"id\":\"B\",\"label\":\"B\",\"type\":\"foundation.thermal_liquid.thermal_liquid\"}],\"Top\":[]}"
  Controlled Heat Flow Rate Source : fl_lib/Thermal/Thermal Sources/Controlled Heat Flow Rate Source
      settings: LogSimulationData=on
  Convective Heat Transfer : fl_lib/Thermal/Thermal Elements/Convective Heat Transfer  thermal_type=foundation.enum.constant_variable.constant  area=fuelGraphiteArea/N_nodes m^2  heat_tr_coeff=fuelGraphiteHeatTransferCoefficient W/(K*m^2)  min_heat_tr_coeff=1e-3 W/(K*m^2)  T_specify=off  T_priority=None  T=0 K  T_nominal_specify=off  T_nominal_value=1  T_nominal_unit=K  Q_specify=off  Q_priority=None  Q=0 W  Q_nominal_specify=off  Q_nominal_value=1  Q_nominal_unit=W
  Fuel Deposited : fl_lib/Physical Signals/Functions/PS Gain  gain=FuelDepositRatio*CoreVolume*axialPowerFraction(3) m^3
  Grahite Deposited : fl_lib/Thermal/Thermal Sources/Controlled Heat Flow Rate Source
      settings: LogSimulationData=on
  Graphite Deposited : fl_lib/Physical Signals/Functions/PS Gain  gain=(1-FuelDepositRatio)*CoreVolume*axialPowerFraction(3) m^3
  Gravity : Subsystem
  Local Resistance (TL) : SimscapeFluids_lib/Thermal Liquid/Pipes & Fittings/Local Resistance (TL)  resistance_loss_spec=fluids.thermal_liquid.pipes_fittings.enum.ResistanceLossSpec.Constant  loss_coeff_AB=fuelChannelLength/N_nodes/fuelChannelHydrualicDiameter*0.07  loss_coeff_BA=fuelChannelLength/N_nodes/fuelChannelHydrualicDiameter*0.07  Re_TLU=[-500, -200, -100, -50, -40, -30, -20, -10, 10, 20, 30, 40, 50, 100, 200, 500, 1000, 2000]  loss_coeff_TLU=[.65, .75, .9, 1.15, 1.35, 1.65, 2.3, 3.1, 4, 2.7, 1.8, 1.46, 1.3, .9, .65, .42, .3, .2]  flow_area=coreFlowArea m^2  Re_c=150
      settings: InternalSimscapePortConfiguration="{\"Bottom\":[],\"Left\":[{\"id\":\"A\",\"label\":\"A\",\"type\":\"foundation.thermal_liquid.thermal_liquid\"}],\"Right\":[{\"id\":\"B\",\"label\":\"B\",\"type\":\"foundation.thermal_liquid.thermal_liquid\"}],\"Top\":[]}"
  Temperature Sensor : fl_lib/Thermal/Thermal Sensors/Temperature Sensor  temperature_measure=foundation.enum.MeasurementReference.difference
  Temperature Sensor1 : fl_lib/Thermal/Thermal Sensors/Temperature Sensor  temperature_measure=foundation.enum.MeasurementReference.difference
  Thermal Mass : fl_lib/Thermal/Thermal Elements/Thermal Mass  mass_type=foundation.enum.constant_variable.constant  mass=CoreVolume*(1-FuelFraction)*rho_graphite/N_nodes kg  sp_heat=cp_graphite J/(K*kg)  mass_min=1e-6 kg  num_ports=foundation.enum.numPorts2.one  m_specify=off  m_priority=High  m=1 kg  m_nominal_specify=off  m_nominal_value=1  m_nominal_unit=kg  T_specify=on  T_priority=High  T=T0 K  T_nominal_specify=off  T_nominal_value=1  T_nominal_unit=K  Q_specify=off  Q_priority=None  Q=0 W  Q_nominal_specify=off  Q_nominal_value=1  Q_nominal_unit=W
      settings: LogSimulationData=on
  Thermal Reference{,1..3} (4 alike) : fl_lib/Thermal/Thermal Elements/Thermal Reference
  Inlet : PMIOPort  Side=Left
  GraphiteA : PMIOPort  Port=2  Side=Left
  PowerDensity : PMIOPort  Port=3  Side=Left
  Outlet : PMIOPort  Port=4  Side=Right
  GraphiteB : PMIOPort  Port=5  Side=Right
  FuelTemp : PMIOPort  Port=6  Side=Right
  GraphiteTemp : PMIOPort  Port=7  Side=Right
  wires:
  GasRef/1 -> 2PModification/1
  connections:
  Grahite Deposited/LConn1 -- Conductive Heat Transfer3/RConn1 -- Conductive Heat Transfer2/RConn1 -- Thermal Mass/LConn1 -- Conductive Heat Transfer1/LConn1
  Graphite Deposited/LConn1 -- Fuel Deposited/LConn1 -- PowerDensity/RConn1
  GraphiteB/RConn1 -- Conductive Heat Transfer1/RConn1 -- Temperature Sensor1/LConn1
  Grahite Deposited/RConn1 -- Graphite Deposited/RConn1
  GraphiteA/RConn1 -- Conductive Heat Transfer2/LConn1
  Controlled Heat Flow Rate Source/RConn2 -- Thermal Reference/LConn1
  Grahite Deposited/RConn2 -- Thermal Reference1/LConn1
  Fuel Deposited/RConn1 -- Controlled Heat Flow Rate Source/RConn1
  Outlet/RConn1 -- 2PModification/RConn1
  Temperature Sensor/RConn1 -- Thermal Reference2/LConn1
  Temperature Sensor/RConn2 -- FuelTemp/RConn1
  2PModification/LConn2 -- Constant Volume Chamber (TL)/RConn1 -- Local Resistance (TL)/LConn1
  Inlet/RConn1 -- Constant Volume Chamber (TL)/LConn1
  2PModification/RConn2 -- 2PModification/LConn1 -- Gravity/RConn1
  Conductive Heat Transfer3/LConn1 -- Convective Heat Transfer/RConn1
  Convective Heat Transfer/LConn1 -- Constant Volume Chamber (TL)/LConn2 -- Temperature Sensor/LConn1 -- Controlled Heat Flow Rate Source/LConn1
  Temperature Sensor1/RConn2 -- GraphiteTemp/RConn1
  Temperature Sensor1/RConn1 -- Thermal Reference3/LConn1
  Gravity/LConn1 -- Local Resistance (TL)/RConn1

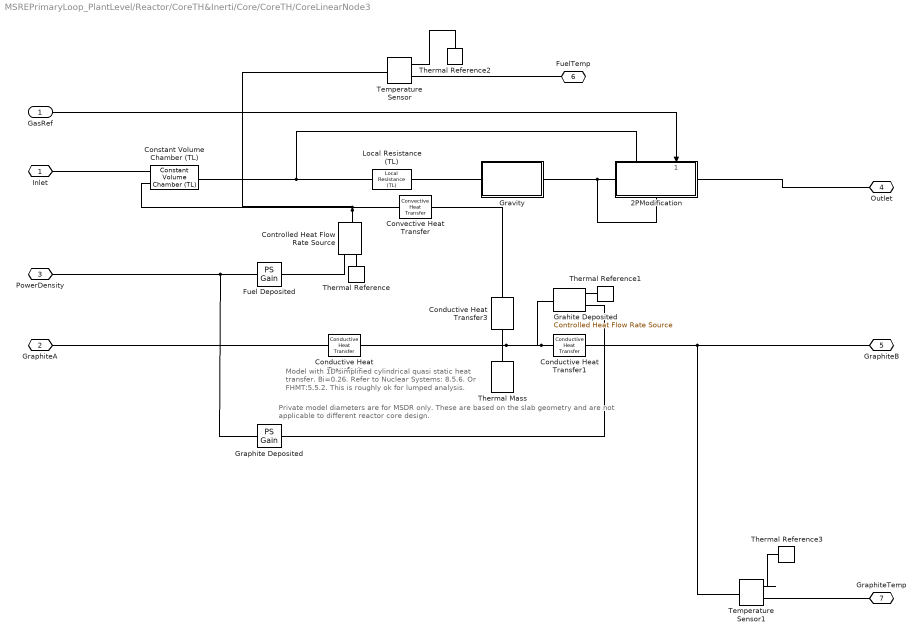
== system MSREPrimaryLoop_PlantLevel/Reactor/CoreTH&Inerti/Core/CoreTH/CoreLinearNode3 ==
  note: Model with 1D simplified cylindrical quasi static heat transfer. Bi=0.26.
      | Refer to Nuclear Systems: 8.5.6. Or FHMT:5.5.2.
      | This is roughly ok for lumped analysis.
  note: Private model diameters are for MSDR only. These are based on the slab geometry and are not applicable to different reactor core design.
  GasRef : Inport
  2PModification : Subsystem  ReferencedSubsystem=TwoPhaseModification
      settings: PortSchema="{\"entries\":[{\"content\":{\"sides\":[{\"content\":{\"connectorIds\":[\"LConn1\"]},\"type\":\"ConnectorPlacement.EquallySpacedRectSide\",\"uuid\":\"7546b4b7-b669-49c8-8f27-f696391ea3ad\"},{\"content\":{\"connectorIds\":[\"RConn1\"],\"side\":\"RIGHT\"},\"type\":\"ConnectorPlacement.EquallySpacedRectSide\",\"uuid\":\"0e6176f2-177c-4327-bcfa-9a190fe9083f\"},{\"content\":{\"connectorIds\":[\"LConn2\",\"In1\"],\"side\":\"TOP\"},\"type\":\"ConnectorPlacement.EquallySpacedRectSide\",\"uuid\":\"16faf74c-4635-4009-a5b3-33dd03b625c6\"},{\"content\":{\"connectorIds\":[\"RConn2\"],\"side\":\"BOTTOM\"},\"type\":\"ConnectorPlacement.EquallySpacedRectSide\",\"uuid\":\"2081d73b-bb08-4ad9-b5c8-e48a4e9c4e20\"}]},\"type\":\"ConnectorPlacement.EquallySpacedConnector\",\"uuid\":\"243e4075-206b-4747-a8bc-b8f10d9a577f\"}],\"packageUris\":[\"http://schema.mathworks.com/mf0/Connector/R2020b\"],\"version\":\"1.0\"}"
  Conductive Heat Transfer1 : fl_lib/Thermal/Thermal Elements/Conductive Heat Transfer  thermal_type=foundation.enum.ConstantVariableTabulated.Constant  wall_geometry=foundation.enum.ConductionWallGeometry.Planar  area=CoreVolume/CoreLength*(1-FuelFraction) m^2  thickness=0.5*CoreLength/N_nodes m  d_in=0.05 m  d_out=0.1 m  L=1 m  th_cond_min=10 W/(K*m)  th_cond=k_graphite W/(m*K)  th_cond_TLU=[413, 401, 392, 383, 371, 357, 342] W/(K*m)  temp_TLU=[200, 273, 400, 600, 800, 1000, 1200] K  T_specify=off  T_priority=None  T=0 K  T_nominal_specify=off  T_nominal_value=1  T_nominal_unit=K  Q_specify=off  Q_priority=None  Q=0 W  Q_nominal_specify=off  Q_nominal_value=1  Q_nominal_unit=W
  Conductive Heat Transfer2 : fl_lib/Thermal/Thermal Elements/Conductive Heat Transfer  thermal_type=foundation.enum.ConstantVariableTabulated.Constant  wall_geometry=foundation.enum.ConductionWallGeometry.Planar  area=CoreVolume/CoreLength*(1-FuelFraction) m^2  thickness=0.5*CoreLength/N_nodes m  d_in=0.05 m  d_out=0.1 m  L=1 m  th_cond_min=10 W/(K*m)  th_cond=k_graphite W/(m*K)  th_cond_TLU=[413, 401, 392, 383, 371, 357, 342] W/(K*m)  temp_TLU=[200, 273, 400, 600, 800, 1000, 1200] K  T_specify=off  T_priority=None  T=0 K  T_nominal_specify=off  T_nominal_value=1  T_nominal_unit=K  Q_specify=off  Q_priority=None  Q=0 W  Q_nominal_specify=off  Q_nominal_value=1  Q_nominal_unit=W
  Conductive Heat Transfer3 : fl_lib/Thermal/Thermal Elements/Conductive Heat Transfer  thermal_type=foundation.enum.ConstantVariableTabulated.Constant  wall_geometry=foundation.enum.ConductionWallGeometry.Planar  area=FuelGraphiteArea/N_nodes m^2  thickness=0.5*UnitCellGraphiteThickness m  d_in=0.05 m  d_out=0.1 m  L=1 m  th_cond_min=10 W/(K*m)  th_cond=k_graphite W/(m*K)  th_cond_TLU=[413, 401, 392, 383, 371, 357, 342] W/(K*m)  temp_TLU=[200, 273, 400, 600, 800, 1000, 1200] K  T_specify=off  T_priority=None  T=0 K  T_nominal_specify=off  T_nominal_value=1  T_nominal_unit=K  Q_specify=off  Q_priority=None  Q=0 W  Q_nominal_specify=off  Q_nominal_value=1  Q_nominal_unit=W
  Constant Volume Chamber (TL) : fl_lib/Thermal Liquid/Elements/Constant Volume Chamber (TL)  volume=coreFuelVolume/N_nodes m^3  num_ports=foundation.enum.num_ports.two  area_A=coreFlowArea m^2  area_B=coreFlowArea m^2  area_C=0.01 m^2  area_D=0.01 m^2  p_I_specify=on  p_I_priority=None  p_I=P0 Pa  p_I_nominal_specify=off  p_I_nominal_value=1  p_I_nominal_unit=MPa  T_I_specify=on  T_I_priority=None  T_I=T0 K  T_I_nominal_specify=on  T_I_nominal_value=T0  T_I_nominal_unit=K  u_I_specify=on  u_I_priority=None  u_I=cpMSRE J/kg  u_I_nominal_specify=off  u_I_nominal_value=1  u_I_nominal_unit=kJ/kg  rho_I_specify=on  rho_I_priority=None  rho_I=nominalFuelDensity kg/m^3  rho_I_nominal_specify=off  rho_I_nominal_value=1  rho_I_nominal_unit=kg/m^3
      settings: LogSimulationData=on  InternalSimscapePortConfiguration="{\"Bottom\":[],\"Left\":[{\"id\":\"A\",\"label\":\"A\",\"type\":\"foundation.thermal_liquid.thermal_liquid\"},{\"id\":\"H\",\"label\":\"H\",\"type\":\"foundation.thermal.thermal\"}],\"Right\":[{\"id\":\"B\",\"label\":\"B\",\"type\":\"foundation.thermal_liquid.thermal_liquid\"}],\"Top\":[]}"
  Controlled Heat Flow Rate Source : fl_lib/Thermal/Thermal Sources/Controlled Heat Flow Rate Source
      settings: LogSimulationData=on
  Convective Heat Transfer : fl_lib/Thermal/Thermal Elements/Convective Heat Transfer  thermal_type=foundation.enum.constant_variable.constant  area=fuelGraphiteArea/N_nodes m^2  heat_tr_coeff=fuelGraphiteHeatTransferCoefficient W/(K*m^2)  min_heat_tr_coeff=1e-3 W/(K*m^2)  T_specify=off  T_priority=None  T=0 K  T_nominal_specify=off  T_nominal_value=1  T_nominal_unit=K  Q_specify=off  Q_priority=None  Q=0 W  Q_nominal_specify=off  Q_nominal_value=1  Q_nominal_unit=W
  Fuel Deposited : fl_lib/Physical Signals/Functions/PS Gain  gain=FuelDepositRatio*CoreVolume*axialPowerFraction(4) m^3
  Grahite Deposited : fl_lib/Thermal/Thermal Sources/Controlled Heat Flow Rate Source
      settings: LogSimulationData=on
  Graphite Deposited : fl_lib/Physical Signals/Functions/PS Gain  gain=(1-FuelDepositRatio)*CoreVolume*axialPowerFraction(4) m^3
  Gravity : Subsystem
  Local Resistance (TL) : SimscapeFluids_lib/Thermal Liquid/Pipes & Fittings/Local Resistance (TL)  resistance_loss_spec=fluids.thermal_liquid.pipes_fittings.enum.ResistanceLossSpec.Constant  loss_coeff_AB=fuelChannelLength/N_nodes/fuelChannelHydrualicDiameter*0.07  loss_coeff_BA=fuelChannelLength/N_nodes/fuelChannelHydrualicDiameter*0.07  Re_TLU=[-500, -200, -100, -50, -40, -30, -20, -10, 10, 20, 30, 40, 50, 100, 200, 500, 1000, 2000]  loss_coeff_TLU=[.65, .75, .9, 1.15, 1.35, 1.65, 2.3, 3.1, 4, 2.7, 1.8, 1.46, 1.3, .9, .65, .42, .3, .2]  flow_area=coreFlowArea m^2  Re_c=150
      settings: InternalSimscapePortConfiguration="{\"Bottom\":[],\"Left\":[{\"id\":\"A\",\"label\":\"A\",\"type\":\"foundation.thermal_liquid.thermal_liquid\"}],\"Right\":[{\"id\":\"B\",\"label\":\"B\",\"type\":\"foundation.thermal_liquid.thermal_liquid\"}],\"Top\":[]}"
  Temperature Sensor : fl_lib/Thermal/Thermal Sensors/Temperature Sensor  temperature_measure=foundation.enum.MeasurementReference.difference
  Temperature Sensor1 : fl_lib/Thermal/Thermal Sensors/Temperature Sensor  temperature_measure=foundation.enum.MeasurementReference.difference
  Thermal Mass : fl_lib/Thermal/Thermal Elements/Thermal Mass  mass_type=foundation.enum.constant_variable.constant  mass=CoreVolume*(1-FuelFraction)*rho_graphite/N_nodes kg  sp_heat=cp_graphite J/(K*kg)  mass_min=1e-6 kg  num_ports=foundation.enum.numPorts2.one  m_specify=off  m_priority=High  m=1 kg  m_nominal_specify=off  m_nominal_value=1  m_nominal_unit=kg  T_specify=on  T_priority=High  T=T0 K  T_nominal_specify=off  T_nominal_value=1  T_nominal_unit=K  Q_specify=off  Q_priority=None  Q=0 W  Q_nominal_specify=off  Q_nominal_value=1  Q_nominal_unit=W
      settings: LogSimulationData=on
  Thermal Reference{,1..3} (4 alike) : fl_lib/Thermal/Thermal Elements/Thermal Reference
  Inlet : PMIOPort  Side=Left
  GraphiteA : PMIOPort  Port=2  Side=Left
  PowerDensity : PMIOPort  Port=3  Side=Left
  Outlet : PMIOPort  Port=4  Side=Right
  GraphiteB : PMIOPort  Port=5  Side=Right
  FuelTemp : PMIOPort  Port=6  Side=Right
  GraphiteTemp : PMIOPort  Port=7  Side=Right
  wires:
  GasRef/1 -> 2PModification/1
  connections:
  Temperature Sensor1/RConn1 -- Thermal Reference3/LConn1
  Temperature Sensor1/RConn2 -- GraphiteTemp/RConn1
  Conductive Heat Transfer3/LConn1 -- Convective Heat Transfer/RConn1
  Gravity/LConn1 -- Local Resistance (TL)/RConn1
  Inlet/RConn1 -- Constant Volume Chamber (TL)/LConn1
  Local Resistance (TL)/LConn1 -- Constant Volume Chamber (TL)/RConn1 -- 2PModification/LConn2
  Temperature Sensor/RConn2 -- FuelTemp/RConn1
  Temperature Sensor/RConn1 -- Thermal Reference2/LConn1
  Fuel Deposited/RConn1 -- Controlled Heat Flow Rate Source/RConn1
  Grahite Deposited/RConn2 -- Thermal Reference1/LConn1
  Controlled Heat Flow Rate Source/RConn2 -- Thermal Reference/LConn1
  GraphiteA/RConn1 -- Conductive Heat Transfer2/LConn1
  Grahite Deposited/RConn1 -- Graphite Deposited/RConn1
  Temperature Sensor1/LConn1 -- Conductive Heat Transfer1/RConn1 -- GraphiteB/RConn1
  PowerDensity/RConn1 -- Fuel Deposited/LConn1 -- Graphite Deposited/LConn1
  Conductive Heat Transfer1/LConn1 -- Thermal Mass/LConn1 -- Conductive Heat Transfer2/RConn1 -- Conductive Heat Transfer3/RConn1 -- Grahite Deposited/LConn1
  2PModification/LConn1 -- Gravity/RConn1 -- 2PModification/RConn2
  Controlled Heat Flow Rate Source/LConn1 -- Temperature Sensor/LConn1 -- Constant Volume Chamber (TL)/LConn2 -- Convective Heat Transfer/LConn1
  2PModification/RConn1 -- Outlet/RConn1

== system MSREPrimaryLoop_PlantLevel/Reactor/CoreTH&Inerti/Core/CoreTH/PowerDensity ==
  note: This is a bit weird as the decay power is part of the total power.
      | I need to check the ratio of total power to decay power.
      | A few percent, not a huge deal for normal operation I suppose?
      | 5% on a log plot. Potentially a peak at 1/160 *2*pi~0.04.
  DecayFraction : Inport
  NeutronFraction : Inport  Port=2
  DecayPowerDensity : fl_lib/Physical Signals/Sources/PS Constant  constant=ReactorPower/CoreVolume*FuelInCoreRatio W/m^3
  PS Gain : fl_lib/Physical Signals/Functions/PS Gain  gain=3
  PS Min : fl_lib/Physical Signals/Nonlinear Operators/PS Min
      settings: InternalSimscapePortConfiguration="{\"Bottom\":[],\"Left\":[{\"id\":\"I1\",\"label\":\"\",\"type\":\"input\"},{\"id\":\"I2\",\"label\":\"\",\"type\":\"input\"}],\"Right\":[{\"id\":\"O\",\"label\":\"\",\"type\":\"output\"}],\"Top\":[]}"
  PS Product : fl_lib/Physical Signals/Functions/PS Product
  PS Product1 : fl_lib/Physical Signals/Functions/PS Product
  PowerDensity : fl_lib/Physical Signals/Sources/PS Constant  constant=ReactorPower*(1-decaySSFraction)/CoreVolume W/m^3
  Simulink-PS Converter : nesl_utility/Simulink-PS Converter  PhysicalDomain=network_engine_domain  SubClassName=ps_input  LeftPortType=input  RightPortType=output  PseudoPeriodic=off  Frequencies=[]  NoiseDistribution=none  NoiseParameters=[]  Unit=1  AffineConversion=off  FilteringAndDerivatives=provide  SimscapeFilterOrder=1  InputFilterTimeConstant=0.001  UdotUserProvided=0
  Simulink-PS Converter1 : nesl_utility/Simulink-PS Converter  PhysicalDomain=network_engine_domain  SubClassName=ps_input  LeftPortType=input  RightPortType=output  PseudoPeriodic=off  Frequencies=[]  NoiseDistribution=none  NoiseParameters=[]  Unit=1  AffineConversion=off  FilteringAndDerivatives=provide  SimscapeFilterOrder=1  InputFilterTimeConstant=0.001  UdotUserProvided=0
  TotalCorePower : fl_lib/Physical Signals/Functions/PS Add
  Conn1 : PMIOPort  Side=Right
  wires:
  DecayFraction/1 -> Simulink-PS Converter1/1
  NeutronFraction/1 -> Simulink-PS Converter/1
  connections:
  PS Product/RConn1 -- TotalCorePower/LConn1
  TotalCorePower/RConn1 -- PS Min/LConn2
  DecayPowerDensity/RConn1 -- PS Product1/LConn2
  PS Gain/RConn1 -- PS Min/LConn1
  Simulink-PS Converter/RConn1 -- PS Product/LConn2
  Simulink-PS Converter1/RConn1 -- PS Product1/LConn1
  PS Product1/RConn1 -- TotalCorePower/LConn2
  PS Min/RConn1 -- Conn1/RConn1
  PS Product/LConn1 -- PowerDensity/RConn1 -- PS Gain/LConn1
